simulink model "bh_3d_pend_sim_CONTROLLED"  (R2021b)
settings: Solver=ode45  StartTime=0.0  StopTime=25  FixedStep=0.001  RelTol=1e-6  AbsTol=1e-6  EnableMultiTasking=on
values from neighbouring files (symbols this model uses):
  K_LAW = [-78.361088012 1.69049101304e-13 6.50451101042e-15 -1.63175637691e-13 78.361088012 1.28612744558e-13 -17.2276366633 -1.91362461096e-14 -9.31673797735e-15 8.02726907722e-14 -17.2276366633 -2.57973956871e-14 ... (39 elements, 3x13)]    [OLD_bh_CONT_DES_RESULTS.mat]    (also in bh_CONT_DES_RESULTS.mat = [-78.361088012 -5.38759787414e-13 -4.00721571005e-14 3.64954)
undefined symbols (not defined in the file or in its folder): DOT_Phi_Theta_Psi, DOT_XYZ, g, Hx, Hy, Hz, Lx, Ly, Lz, M_cart, m_pend, Phi_Theta_Psi, q0_ang_deg, q0_dot_and_deg, sigbuilder_block, X, XYZ, Y, Z
libraries: nesl_utility x14, simulink_extras x11, sm_lib x9
(part 1 of 2)
settings Model: Creator=bhorton  LastModifiedBy=bhorton
settings SolverCC: ZeroCrossAlgorithm=Adaptive  AlgebraicLoopSolver=TrustRegion
settings DataIOCC: LimitDataPoints=on  ReturnWorkspaceOutputs=off
settings OptimizationCC: LifeSpan=inf
settings DebuggingCC: AllowSymbolicDim=off  PregeneratedLibrarySubsystemCodeDiagnostic=none  SFUnexpectedBacktrackingDiag=warning  SFNoUnconditionalDefaultTransitionDiag=warning  SFExecutionAtInitializationDiag=none  SFMachineParentedDataDiag=warning  ArithmeticOperatorsInVariantConditions=warning
settings SFSimCC: SimUseLocalCustomCode=off  CustomCodeUndefinedFunction=UseInterfaceOnly
settings RTWCC: RTWUseLocalCustomCode=off
settings CodeAppCC: StateflowObjectComments=on
settings GRTTargetCC: TargetLangStandard=C89/C90 (ANSI)
settings ConfigComp: CovMetricSettings=dw  CovSaveCumulativeToWorkspaceVar=on  CovSaveSingleToWorkspaceVar=on  CovExternalEMLEnable=off  CovSFcnEnable=off
settings SimscapeCC: SimscapeNormalizeSystem=off  SimscapeLogType=all  SimscapeLogDataHistory=10000
settings ConfigurationSet: Description=SimMechanics 2G
settings ExplorerConfigSet: InternalSimMechanicsExplorerSettings="<ExplorerConfiguration><canonicalview>default</canonicalview><AnimationSetting><BasePlaybackSpeed>1.0</BasePlaybackSpeed><PlaybackSpeedFactor>1.0</PlaybackSpeedFactor></AnimationSetting><TilePanel><TileInfo><Tiles Columns=\"2\" Count=\"4\" Rows=\"2\"><Column Left=\"2\" Weight=\"0.4993\"/><Column Left=\"299\" Weight=\"0.5007\"/><Column Left=\"596\"/><Row Top=\"2\" Weight=\"0.4991\"/><Row Top=\"230\" Weight=\"0.5009\"/><Row Top=\"459\"/><Tile Height=\"1\" Width=\"1\" X=\"0\" Y=\"0\"/><Tile Height=\"1\" Width=\"1\" X=\"0\" Y=\"1\"/><Tile Height=\"1\" Width=\"1\" X=\"1\" Y=\"0\"/><Tile Height=\"1\" Width=\"1\" X=\"1\" Y=\"1\"/></Tiles></TileInfo><SceneInfo><SceneViewer><BGColor><R>0.60000002384185791</R><G>0.60000002384185791</G><B>0.60000002384185791</B></BGColor><Camera><DoPerspective>off</DoPerspective><Position><X>0.0066101237906532632</X><Y>-1.0000000187716092</Y><Z>0.27830506136231026</Z></Position><Center><X>0.0066101237906532632</X><Y>-1.8771609211487572e-08</Y><Z>0.27830506136231026</Z></Center><Up><X>0</X><Y>-0</Y><Z>1</Z></Up><ViewLimDist>1</ViewLimDist><YLim>0.6337593571276271</YLim><XLim>0.8334369627979753</XLim></Camera></SceneViewer><SceneViewer><BGColor><R>0.60000002384185791</R><G>0.60000002384185791</G><B>0.60000002384185791</B></BGColor><Camera><DoPerspective>off</DoPerspective><Position><X>0.12097194898226168</X><Y>-0.1831262202380439</Y><Z>1.2750000010896152</Z></Position><Center><X>0.12097194898226168</X><Y>-0.1831262202380439</Y><Z>0.2750000010896152</Z></Center><Up><X>0</X><Y>1</Y><Z>-0</Z></Up><ViewLimDist>1</ViewLimDist><YLim>0.56280693766119472</YLim><XLim>0.73676544566556401</XLim></Camera></SceneViewer><SceneViewer><BGColor><R>0.60000002384185791</R><G>0.60000002384185791</G><B>0.60000002384185791</B></BGColor><Camera><DoPerspective>off</DoPerspective><Position><X>1.0477103451195624</X><Y>0.043433240975990085</Y><Z>0.24150487446228938</Z></Position><Center><X>3.245263613393945e-09</X><Y>0.043433240975990085</Y><Z>0.24150487446228938</Z></Center><Up><X>-0</X><Y>0</Y><Z>1</Z></Up><ViewLimDist>1</ViewLimDist><YLim>0.53585596018430881</YLim><XLim>0.70468729010539233</XLim></Camera></SceneViewer><SceneViewer><BGColor><R>0.60000002384185791</R><G>0.60000002384185791</G><B>0.60000002384185791</B></BGColor><Camera><DoPerspective>off</DoPerspective><Position><X>0.62223409931486595</X><Y>-0.53029272300920749</Y><Z>0.80202361126646926</Z></Position><Center><X>0.044883830125240165</X><Y>0.047057546180418207</Y><Z>0.2246733420768435</Z></Center><Up><X>-0.40824829046386307</X><Y>0.40824829046386307</Y><Z>0.81649658092772615</Z></Up><ViewLimDist>1</ViewLimDist><YLim>0.76349703631239541</YLim><XLim>0.99948702935440847</XLim></Camera></SceneViewer></SceneInfo></TilePanel><MechEditorPanel><Cameras/><GfxPanelCameraMap/><VideoCreator><PlaybackSpeedRatio>1.0</PlaybackSpeedRatio><FrameRate>30</FrameRate><VideoFormat>Motion JPEG AVI</VideoFormat><FrameSize>auto</FrameSize></VideoCreator></MechEditorPanel></ExplorerConfiguration>"

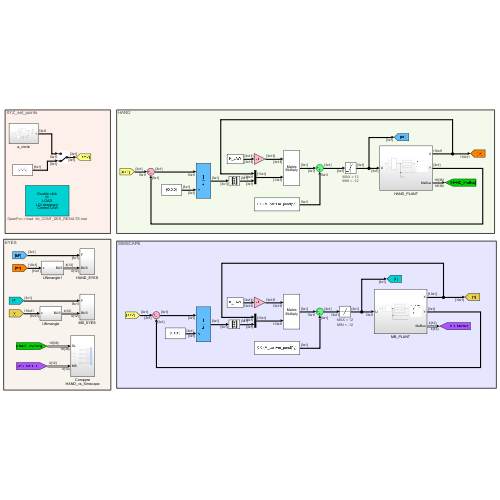
[thumbnail: Simulink's stored preview of the top-level diagram]
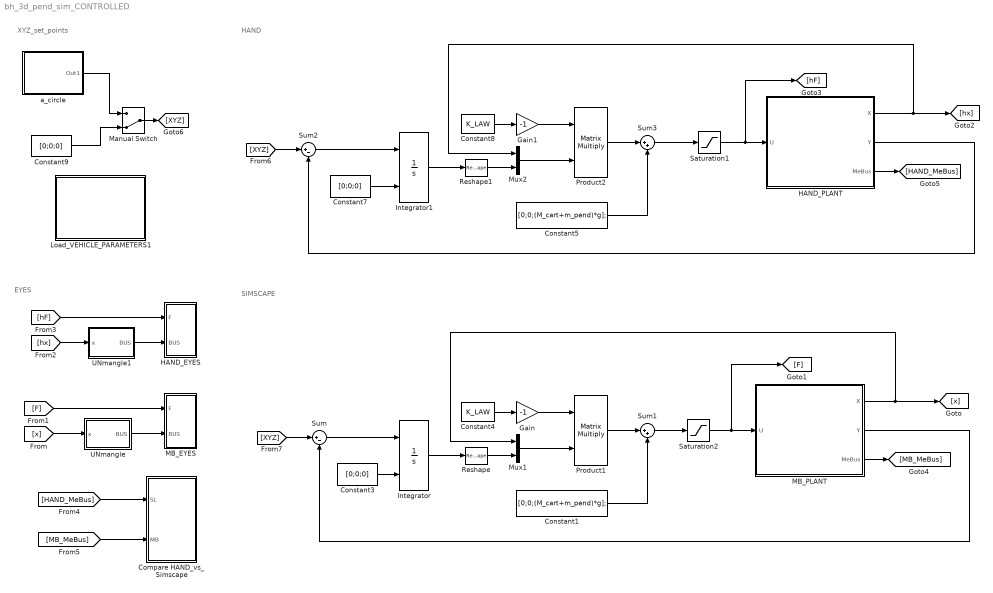
== system bh_3d_pend_sim_CONTROLLED ==
  note: XYZ_set_points
  note: EYES
  note: HAND
  note: SIMSCAPE
  Compare HAND_vs_Simscape : Subsystem
  Constant1 : Constant  Value=[0;0;(M_cart+m_pend)*g];  VectorParams1D=off
  Constant3 : Constant  Value=[0;0;0]  VectorParams1D=off
  Constant4 : Constant  Value=K_LAW  VectorParams1D=off
  Constant5 : Constant  Value=[0;0;(M_cart+m_pend)*g];  VectorParams1D=off
  Constant7 : Constant  Value=[0;0;0]  VectorParams1D=off
  Constant8 : Constant  Value=K_LAW  VectorParams1D=off
  Constant9 : Constant  Value=[0;0;0]  VectorParams1D=off
  Gain : Gain  Gain=-1
  Gain1 : Gain  Gain=-1
  HAND_EYES : Subsystem
  HAND_PLANT : Subsystem
  Integrator : Integrator  InitialConditionSource=external
  Integrator1 : Integrator  InitialConditionSource=external
  Load_VEHICLE_PARAMETERS1 : Subsystem
      settings: AttributesFormatString=OpenFcn = %<OpenFcn>  OpenFcn="load  bh_CONT_DES_RESULTS.mat"
      mask Display: disp('Double click\nto\nLOAD\nLQI designed \n Control LAW')
  MB_EYES : Subsystem
  MB_PLANT : Subsystem
  Manual Switch : ManualSwitch  CurrentSetting=0
  Mux1 : Mux  Inputs=2
  Mux2 : Mux  Inputs=2
  Product1 : Product  Multiplication=Matrix(*)
  Product2 : Product  Multiplication=Matrix(*)
  Reshape : Reshape  OutputDimensionality=Column vector (2-D)
  Reshape1 : Reshape  OutputDimensionality=Column vector (2-D)
  Saturation1 : Saturate  UpperLimit=12  LowerLimit=-12
      settings: AttributesFormatString=|
      | MAX = %<UpperLimit>
      | MIN = %<LowerLimit>
  Saturation2 : Saturate  UpperLimit=12  LowerLimit=-12
      settings: AttributesFormatString=|
      | MAX = %<UpperLimit>
      | MIN = %<LowerLimit>
  Sum : Sum  Inputs=|+-
  Sum1 : Sum  Inputs=|++
  Sum2 : Sum  Inputs=|+-
  Sum3 : Sum  Inputs=|++
  UNmangle : Subsystem
  UNmangle1 : Subsystem
  a_circle : Subsystem
  wires:
  Mux1/1 -> Product1/2
  Integrator/1 -> Reshape/1
  MB_PLANT/2(Y) -> Sum/2
  Constant3/1 -> Integrator/2
  Product1/1 -> Sum1/1
  Gain/1 -> Product1/1
  Sum/1 -> Integrator/1
  MB_PLANT/1(X) -> [x], Mux1/1
  [XYZ] -> Sum/1
  Constant4/1 -> Gain/1
  Reshape/1 -> Mux1/2
  [F] -> MB_EYES/1(F)
  UNmangle/1(BUS) -> MB_EYES/2(BUS)
  [x] -> UNmangle/1(x)
  Saturation2/1 -> [F], MB_PLANT/1(U)
  Sum1/1 -> Saturation2/1
  Constant1/1 -> Sum1/2
  Saturation1/1 -> [hF], HAND_PLANT/1(U)
  Gain1/1 -> Product2/1
  Constant7/1 -> Integrator1/2
  Sum3/1 -> Saturation1/1
  Sum2/1 -> Integrator1/1
  [XYZ] -> Sum2/1
  HAND_PLANT/2(Y) -> Sum2/2
  Mux2/1 -> Product2/2
  Integrator1/1 -> Reshape1/1
  Product2/1 -> Sum3/1
  Reshape1/1 -> Mux2/2
  Constant5/1 -> Sum3/2
  Constant8/1 -> Gain1/1
  HAND_PLANT/1(X) -> [hx], Mux2/1
  UNmangle1/1(BUS) -> HAND_EYES/2(BUS)
  [hx] -> UNmangle1/1(x)
  [hF] -> HAND_EYES/1(F)
  [HAND_MeBus] -> Compare HAND_vs_Simscape/1(SL)
  [MB_MeBus] -> Compare HAND_vs_Simscape/2(MB)
  HAND_PLANT/3(MeBus) -> [HAND_MeBus]
  MB_PLANT/3(MeBus) -> [MB_MeBus]
  a_circle/1(Out1) -> Manual Switch/1
  Constant9/1 -> Manual Switch/2
  Manual Switch/1 -> [XYZ]

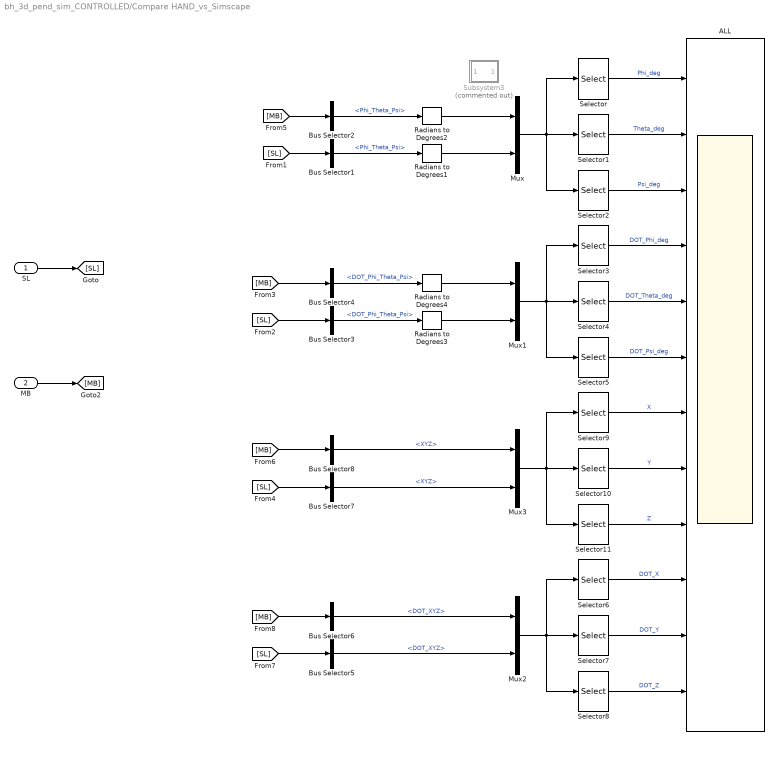
== system bh_3d_pend_sim_CONTROLLED/Compare HAND_vs_Simscape ==
  SL : Inport
  MB : Inport  Port=2
  ALL : Scope  NumInputPorts=12
  Bus Selector1 : BusSelector  OutputSignals=Phi_Theta_Psi
  Bus Selector2 : BusSelector  OutputSignals=Phi_Theta_Psi
  Bus Selector3 : BusSelector  OutputSignals=DOT_Phi_Theta_Psi
  Bus Selector4 : BusSelector  OutputSignals=DOT_Phi_Theta_Psi
  Bus Selector5 : BusSelector  OutputSignals=DOT_XYZ
  Bus Selector6 : BusSelector  OutputSignals=DOT_XYZ
  Bus Selector7 : BusSelector  OutputSignals=XYZ
  Bus Selector8 : BusSelector  OutputSignals=XYZ
  Mux{,1..3} (4 alike) : Mux  Inputs=2
  Radians to Degrees{1..4} (4 alike) : simulink_extras/Transformations/Radians to Degrees
  Selector{,3,6,9} (4 alike) : Selector  InputPortWidth=6  IndexOptions=Index vector (dialog)  Indices=[1 4]  OutputSizes=1
  Selector{1,4,7,10} (4 alike) : Selector  InputPortWidth=6  IndexOptions=Index vector (dialog)  Indices=[2 5]  OutputSizes=1
  Selector{2,5,8,11} (4 alike) : Selector  InputPortWidth=6  IndexOptions=Index vector (dialog)  Indices=[3 6]  OutputSizes=1
  Subsystem3 : Subsystem  Commented=on
      mask Display: disp(sprintf('Mod\n360'))
  wires:
  SL/1 -> [SL]
  MB/1 -> [MB]
  Bus Selector1/1 -> Radians to Degrees1/1  "<Phi_Theta_Psi>"
  Bus Selector2/1 -> Radians to Degrees2/1  "<Phi_Theta_Psi>"
  Radians to Degrees1/1 -> Mux/2
  Radians to Degrees2/1 -> Mux/1
  Selector/1 -> ALL/1  "Phi_deg"
  Selector2/1 -> ALL/3  "Psi_deg"
  Selector1/1 -> ALL/2  "Theta_deg"
  Mux/1 -> Selector2/1, Selector/1, Selector1/1
  Bus Selector3/1 -> Radians to Degrees3/1  "<DOT_Phi_Theta_Psi>"
  Radians to Degrees3/1 -> Mux1/2
  Bus Selector4/1 -> Radians to Degrees4/1  "<DOT_Phi_Theta_Psi>"
  Radians to Degrees4/1 -> Mux1/1
  Mux1/1 -> Selector5/1, Selector3/1, Selector4/1
  Selector4/1 -> ALL/5  "DOT_Theta_deg"
  Selector3/1 -> ALL/4  "DOT_Phi_deg"
  Selector5/1 -> ALL/6  "DOT_Psi_deg"
  Mux2/1 -> Selector8/1, Selector6/1, Selector7/1
  Bus Selector6/1 -> Mux2/1  "<DOT_XYZ>"
  Bus Selector5/1 -> Mux2/2  "<DOT_XYZ>"
  Selector7/1 -> ALL/11  "DOT_Y"
  Selector8/1 -> ALL/12  "DOT_Z"
  Selector6/1 -> ALL/10  "DOT_X"
  Bus Selector7/1 -> Mux3/2  "<XYZ>"
  Bus Selector8/1 -> Mux3/1  "<XYZ>"
  Mux3/1 -> Selector11/1, Selector9/1, Selector10/1
  Selector9/1 -> ALL/7  "X"
  Selector10/1 -> ALL/8  "Y"
  Selector11/1 -> ALL/9  "Z"
  [MB] -> Bus Selector2/1
  [SL] -> Bus Selector1/1
  [MB] -> Bus Selector6/1
  [SL] -> Bus Selector5/1
  [SL] -> Bus Selector7/1
  [MB] -> Bus Selector8/1
  [SL] -> Bus Selector3/1
  [MB] -> Bus Selector4/1

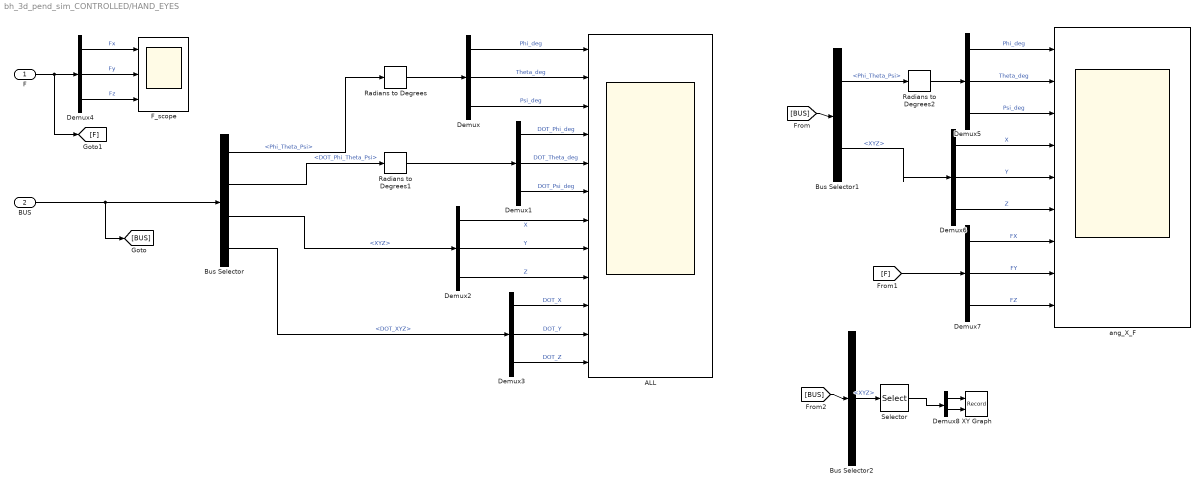
== system bh_3d_pend_sim_CONTROLLED/HAND_EYES ==
  F : Inport
  BUS : Inport  Port=2
  ALL : Scope  NumInputPorts=12
  Bus Selector : BusSelector  OutputSignals=Phi_Theta_Psi,DOT_Phi_Theta_Psi,XYZ,DOT_XYZ
  Bus Selector1 : BusSelector  OutputSignals=Phi_Theta_Psi,XYZ
  Bus Selector2 : BusSelector  OutputSignals=XYZ
  Demux{,1..7} (8 alike) : Demux  Outputs=3
  Demux8 : Demux  Outputs=2
  F_scope : Scope  NumInputPorts=3
  Radians to Degrees : simulink_extras/Transformations/Radians to Degrees
  Radians to Degrees1 : simulink_extras/Transformations/Radians to Degrees
  Radians to Degrees2 : simulink_extras/Transformations/Radians to Degrees
  Selector : Selector  InputPortWidth=3  IndexOptions=Index vector (dialog)  Indices=[1 2]  OutputSizes=1
  XY Graph : Record  FileSettingsInternal="{\"entries\":[{\"content\":{\"excelSettings\":{\"content\":{},\"type\":\"Streamout.ExcelSettings\"}},\"type\":\"Streamout.FileSettingStorage\",\"uuid\":\"99c117ed-58ae-4b65-b485-cface1eea5be\"}],\"packageUris\":[\"http://schema.mathworks.com/mf0/streamout_blocks/R2020a\"],\"version\":\"1.0\"}"  Layout=[1 1]  SignalsInternal="{\"entries\":[{\"content\":{\"signals\":[{\"content\":{\"blockPath\":[\"bh_3d_pend_sim_CONTROLLED/HAND_EYES/XY Graph\"],\"channel\":[],\"dimensions\":[1,1],\"domain\":\"bh_3d_pend_sim_CONTROLLED/HAND_EYES/XY Graph\",\"lineColor\":\"#a2142f\",\"plots\":[1],\"port\":1,\"sid\":[\"\"],\"signalID\":34,\"signalName\":\"Demux8:1\"},\"type\":\"RecordBlkView.Signal\",\"uuid\":\"b9760cf6-ac66-4326-8e3b-6ee9031ad026\"},{\"content\":{\"blockPath\":[\"bh_3d_pend_sim_CONTROLLED/HAND_EYES/XY Graph\"],\"channel\":[],\"dimensions\":[1,1],\"domain\":\"bh_3d_pend_sim_CONTROLLED/HAND_EYES/XY Graph\",\"lineColor\":\"#139fff\",\"plots\":[1],\"port\":2,\"sid\":[\"\"],\"signalID\":38,\"signalName\":\"Demux8:2\"},\"type\":\"RecordBlkView.Signal\",\"uuid\":\"94cb77a1-340e-480f-8b2e-a2f08ce9c347\"}]},\"type\":\"RecordBlkView.InputSignals\",\"uuid\":\"3dd7e1b0-0053-45f3-aee9-dc3925895e13\"}],\"packageUris\":[\"http://schema.mathworks.com/mf0/streamout_blocks/R2020a\"],\"version\":\"1.0\"}"  VisualizationBindings="{\"xyplotplugin\":{\"info\":[{\"series\":[{\"bindingParametersList\":[{\"parameter\":\"X-Axis\",\"signalID\":34,\"signalName\":\"Demux8:1\"},{\"parameter\":\"Y-Axis\",\"signalID\":38,\"signalName\":\"Demux8:2\"}],\"seriesID\":54278}],\"subplotID\":1}]}}"  CompatibilityTag=XY  st=-1
  ang_X_F : Scope  NumInputPorts=9
  wires:
  Bus Selector/2 -> Radians to Degrees1/1  "<DOT_Phi_Theta_Psi>"
  Bus Selector/1 -> Radians to Degrees/1  "<Phi_Theta_Psi>"
  Demux4/3 -> F_scope/3  "Fz"
  Demux4/1 -> F_scope/1  "Fx"
  Demux/1 -> ALL/1  "Phi_deg"
  Radians to Degrees1/1 -> Demux1/1
  Demux3/3 -> ALL/12  "DOT_Z"
  Demux1/3 -> ALL/6  "DOT_Psi_deg"
  Bus Selector/3 -> Demux2/1  "<XYZ>"
  Demux3/1 -> ALL/10  "DOT_X"
  Demux2/3 -> ALL/9  "Z"
  Demux3/2 -> ALL/11  "DOT_Y"
  Demux2/2 -> ALL/8  "Y"
  Demux2/1 -> ALL/7  "X"
  Demux1/1 -> ALL/4  "DOT_Phi_deg"
  Demux1/2 -> ALL/5  "DOT_Theta_deg"
  Demux/2 -> ALL/2  "Theta_deg"
  BUS/1 -> [BUS], Bus Selector/1
  Demux/3 -> ALL/3  "Psi_deg"
  Bus Selector/4 -> Demux3/1  "<DOT_XYZ>"
  Radians to Degrees/1 -> Demux/1
  Demux4/2 -> F_scope/2  "Fy"
  F/1 -> [F], Demux4/1
  [BUS] -> Bus Selector1/1
  Bus Selector1/1 -> Radians to Degrees2/1  "<Phi_Theta_Psi>"
  Demux5/3 -> ang_X_F/3  "Psi_deg"
  Demux5/2 -> ang_X_F/2  "Theta_deg"
  Demux5/1 -> ang_X_F/1  "Phi_deg"
  Radians to Degrees2/1 -> Demux5/1
  Demux6/1 -> ang_X_F/4  "X"
  Demux6/2 -> ang_X_F/5  "Y"
  Demux6/3 -> ang_X_F/6  "Z"
  Bus Selector1/2 -> Demux6/1  "<XYZ>"
  Demux7/1 -> ang_X_F/7  "FX"
  Demux7/2 -> ang_X_F/8  "FY"
  [F] -> Demux7/1
  Demux7/3 -> ang_X_F/9  "FZ"
  [BUS] -> Bus Selector2/1
  Demux8/1 -> XY Graph/1
  Demux8/2 -> XY Graph/2
  Bus Selector2/1 -> Selector/1  "<XYZ>"
  Selector/1 -> Demux8/1

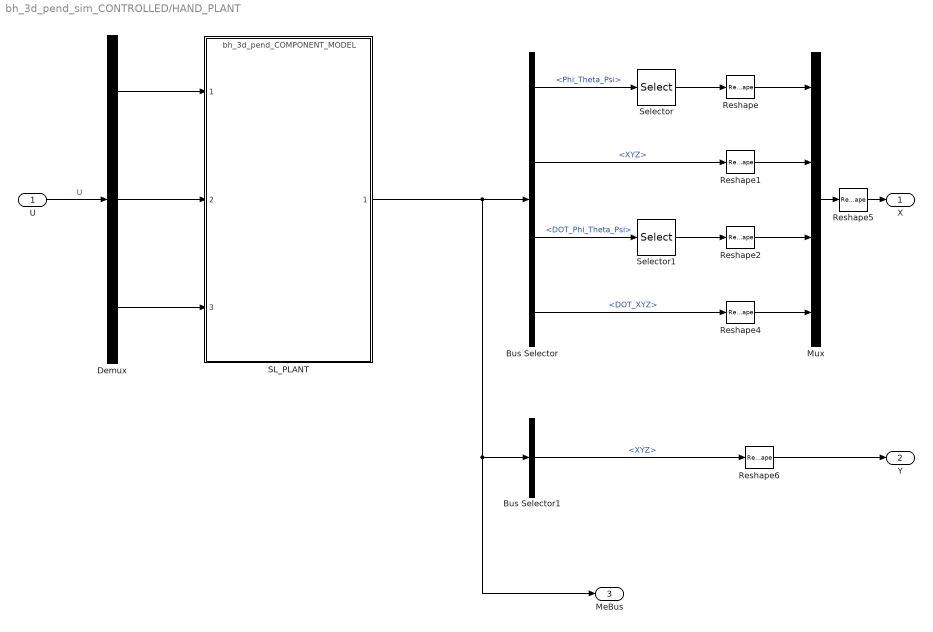
== system bh_3d_pend_sim_CONTROLLED/HAND_PLANT ==
  U : Inport
  Bus Selector : BusSelector  OutputSignals=Phi_Theta_Psi,XYZ,DOT_Phi_Theta_Psi,DOT_XYZ
  Bus Selector1 : BusSelector  OutputSignals=XYZ
  Demux : Demux  Outputs=3
  Mux : Mux
  Reshape{,1..2,4..6} (6 alike) : Reshape  OutputDimensionality=Column vector (2-D)
  SL_PLANT : ModelReference  ModelNameDialog=bh_3d_pend_COMPONENT_MODEL.slx  SimulationMode=Normal  ModelReferenceVersion=5.0
  Selector : Selector  InputPortWidth=3  IndexOptions=Index vector (dialog)  Indices=2:3  OutputSizes=1
  Selector1 : Selector  InputPortWidth=3  IndexOptions=Index vector (dialog)  Indices=2:3  OutputSizes=1
  X : Outport  VectorParamsAs1DForOutWhenUnconnected=off
  Y : Outport  Port=2  VectorParamsAs1DForOutWhenUnconnected=off
  MeBus : Outport  Port=3  VectorParamsAs1DForOutWhenUnconnected=off
  wires:
  Demux/1 -> SL_PLANT/1
  Demux/2 -> SL_PLANT/2
  Demux/3 -> SL_PLANT/3
  U/1 -> Demux/1  "U"
  SL_PLANT/1 -> MeBus/1, Bus Selector1/1, Bus Selector/1
  Bus Selector/1 -> Selector/1  "<Phi_Theta_Psi>"
  Bus Selector/2 -> Reshape1/1  "<XYZ>"
  Bus Selector/3 -> Selector1/1  "<DOT_Phi_Theta_Psi>"
  Selector1/1 -> Reshape2/1
  Selector/1 -> Reshape/1
  Bus Selector/4 -> Reshape4/1  "<DOT_XYZ>"
  Reshape2/1 -> Mux/3
  Reshape1/1 -> Mux/2
  Reshape/1 -> Mux/1
  Reshape4/1 -> Mux/4
  Mux/1 -> Reshape5/1
  Reshape5/1 -> X/1
  Reshape6/1 -> Y/1
  Bus Selector1/1 -> Reshape6/1  "<XYZ>"

== system bh_3d_pend_sim_CONTROLLED/Load_VEHICLE_PARAMETERS1 ==

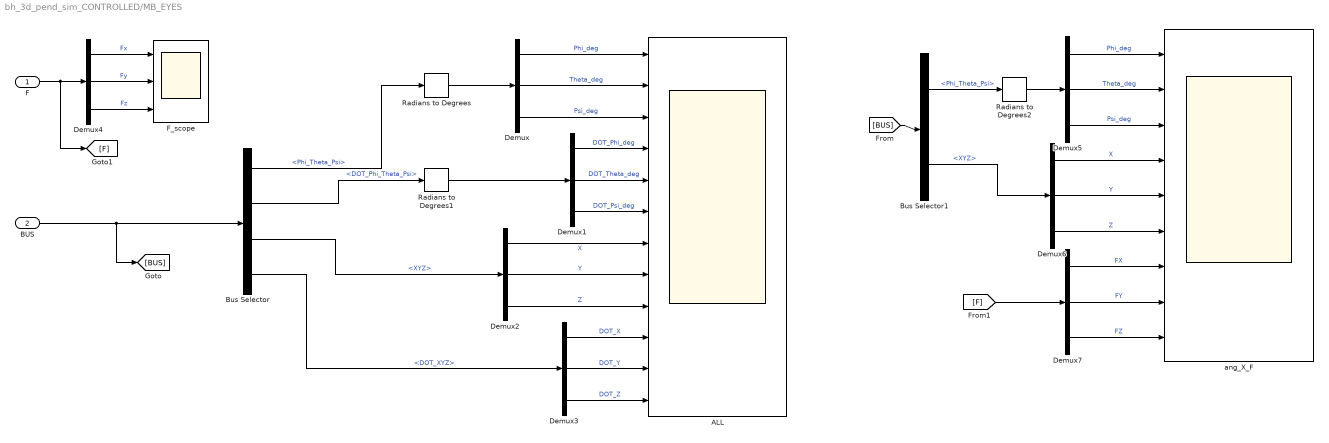
== system bh_3d_pend_sim_CONTROLLED/MB_EYES ==
  F : Inport
  BUS : Inport  Port=2
  ALL : Scope  NumInputPorts=12
  Bus Selector : BusSelector  OutputSignals=Phi_Theta_Psi,DOT_Phi_Theta_Psi,XYZ,DOT_XYZ
  Bus Selector1 : BusSelector  OutputSignals=Phi_Theta_Psi,XYZ
  Demux{,1..7} (8 alike) : Demux  Outputs=3
  F_scope : Scope  NumInputPorts=3
  Radians to Degrees : simulink_extras/Transformations/Radians to Degrees
  Radians to Degrees1 : simulink_extras/Transformations/Radians to Degrees
  Radians to Degrees2 : simulink_extras/Transformations/Radians to Degrees
  ang_X_F : Scope  NumInputPorts=9
  wires:
  Bus Selector/2 -> Radians to Degrees1/1  "<DOT_Phi_Theta_Psi>"
  Bus Selector/1 -> Radians to Degrees/1  "<Phi_Theta_Psi>"
  Demux4/3 -> F_scope/3  "Fz"
  Demux4/1 -> F_scope/1  "Fx"
  Demux/1 -> ALL/1  "Phi_deg"
  Radians to Degrees1/1 -> Demux1/1
  Demux3/3 -> ALL/12  "DOT_Z"
  Demux1/3 -> ALL/6  "DOT_Psi_deg"
  Bus Selector/3 -> Demux2/1  "<XYZ>"
  Demux3/1 -> ALL/10  "DOT_X"
  Demux2/3 -> ALL/9  "Z"
  Demux3/2 -> ALL/11  "DOT_Y"
  Demux2/2 -> ALL/8  "Y"
  Demux2/1 -> ALL/7  "X"
  Demux1/1 -> ALL/4  "DOT_Phi_deg"
  Demux1/2 -> ALL/5  "DOT_Theta_deg"
  Demux/2 -> ALL/2  "Theta_deg"
  BUS/1 -> [BUS], Bus Selector/1
  Demux/3 -> ALL/3  "Psi_deg"
  Bus Selector/4 -> Demux3/1  "<DOT_XYZ>"
  Radians to Degrees/1 -> Demux/1
  Demux4/2 -> F_scope/2  "Fy"
  F/1 -> [F], Demux4/1
  [BUS] -> Bus Selector1/1
  Bus Selector1/1 -> Radians to Degrees2/1  "<Phi_Theta_Psi>"
  Demux5/3 -> ang_X_F/3  "Psi_deg"
  Demux5/2 -> ang_X_F/2  "Theta_deg"
  Demux5/1 -> ang_X_F/1  "Phi_deg"
  Radians to Degrees2/1 -> Demux5/1
  Demux6/1 -> ang_X_F/4  "X"
  Demux6/2 -> ang_X_F/5  "Y"
  Demux6/3 -> ang_X_F/6  "Z"
  Bus Selector1/2 -> Demux6/1  "<XYZ>"
  Demux7/1 -> ang_X_F/7  "FX"
  Demux7/2 -> ang_X_F/8  "FY"
  [F] -> Demux7/1
  Demux7/3 -> ang_X_F/9  "FZ"

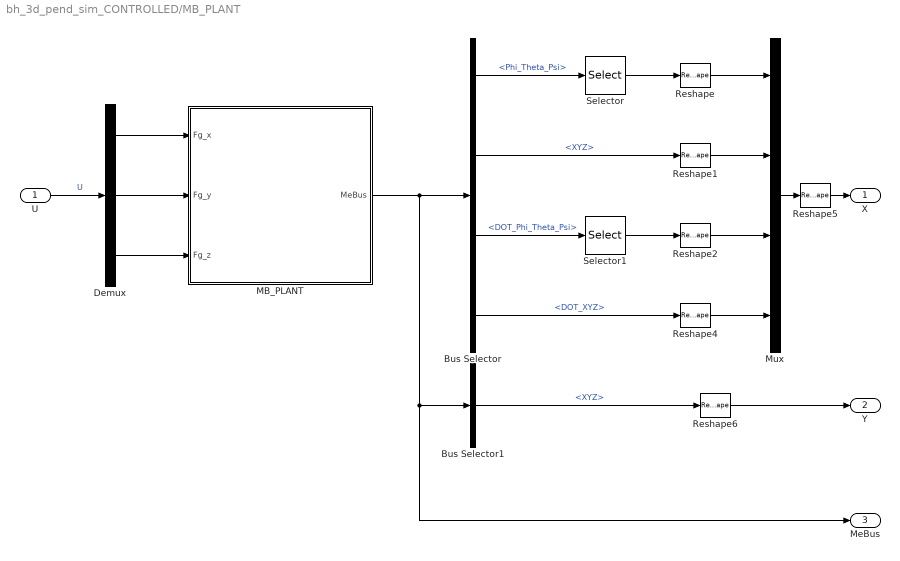
== system bh_3d_pend_sim_CONTROLLED/MB_PLANT ==
  U : Inport
  Bus Selector : BusSelector  OutputSignals=Phi_Theta_Psi,XYZ,DOT_Phi_Theta_Psi,DOT_XYZ
  Bus Selector1 : BusSelector  OutputSignals=XYZ
  Demux : Demux  Outputs=3
  MB_PLANT : Subsystem
  Mux : Mux
  Reshape{,1..2,4..6} (6 alike) : Reshape  OutputDimensionality=Column vector (2-D)
  Selector : Selector  InputPortWidth=3  IndexOptions=Index vector (dialog)  Indices=2:3  OutputSizes=1
  Selector1 : Selector  InputPortWidth=3  IndexOptions=Index vector (dialog)  Indices=2:3  OutputSizes=1
  X : Outport  VectorParamsAs1DForOutWhenUnconnected=off
  Y : Outport  Port=2  VectorParamsAs1DForOutWhenUnconnected=off
  MeBus : Outport  Port=3  VectorParamsAs1DForOutWhenUnconnected=off
  wires:
  Demux/1 -> MB_PLANT/1(Fg_x)
  Demux/2 -> MB_PLANT/2(Fg_y)
  Demux/3 -> MB_PLANT/3(Fg_z)
  U/1 -> Demux/1  "U"
  MB_PLANT/1(MeBus) -> MeBus/1, Bus Selector1/1, Bus Selector/1
  Bus Selector/1 -> Selector/1  "<Phi_Theta_Psi>"
  Bus Selector/2 -> Reshape1/1  "<XYZ>"
  Bus Selector/3 -> Selector1/1  "<DOT_Phi_Theta_Psi>"
  Selector1/1 -> Reshape2/1
  Selector/1 -> Reshape/1
  Bus Selector/4 -> Reshape4/1  "<DOT_XYZ>"
  Reshape2/1 -> Mux/3
  Reshape1/1 -> Mux/2
  Reshape/1 -> Mux/1
  Reshape4/1 -> Mux/4
  Mux/1 -> Reshape5/1
  Reshape5/1 -> X/1
  Reshape6/1 -> Y/1
  Bus Selector1/1 -> Reshape6/1  "<XYZ>"

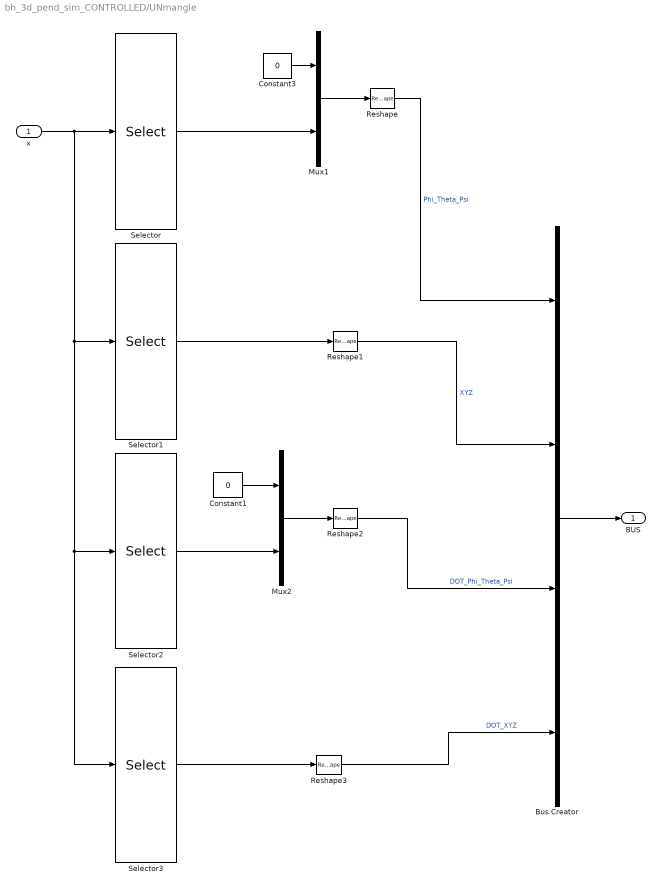
== system bh_3d_pend_sim_CONTROLLED/UNmangle ==
  x : Inport
  Bus Creator : BusCreator  Inputs=4
  Constant1 : Constant  Value=0  VectorParams1D=off
  Constant3 : Constant  Value=0  VectorParams1D=off
  Mux1 : Mux  Inputs=2
  Mux2 : Mux  Inputs=2
  Reshape{,1..3} (4 alike) : Reshape  OutputDimensionality=Column vector (2-D)
  Selector : Selector  InputPortWidth=10  IndexOptions=Index vector (dialog)  Indices=[1,2]  OutputSizes=1
  Selector1 : Selector  InputPortWidth=10  IndexOptions=Index vector (dialog)  Indices=3:5  OutputSizes=1
  Selector2 : Selector  InputPortWidth=10  IndexOptions=Index vector (dialog)  Indices=6:7  OutputSizes=1
  Selector3 : Selector  InputPortWidth=10  IndexOptions=Index vector (dialog)  Indices=8:10  OutputSizes=1
  BUS : Outport  VectorParamsAs1DForOutWhenUnconnected=off
  wires:
  x/1 -> Selector3/1, Selector2/1, Selector1/1, Selector/1
  Constant3/1 -> Mux1/1
  Selector/1 -> Mux1/2
  Mux1/1 -> Reshape/1
  Selector1/1 -> Reshape1/1
  Selector2/1 -> Mux2/2
  Constant1/1 -> Mux2/1
  Mux2/1 -> Reshape2/1
  Selector3/1 -> Reshape3/1
  Bus Creator/1 -> BUS/1
  Reshape/1 -> Bus Creator/1  "Phi_Theta_Psi"
  Reshape1/1 -> Bus Creator/2  "XYZ"
  Reshape2/1 -> Bus Creator/3  "DOT_Phi_Theta_Psi"
  Reshape3/1 -> Bus Creator/4  "DOT_XYZ"

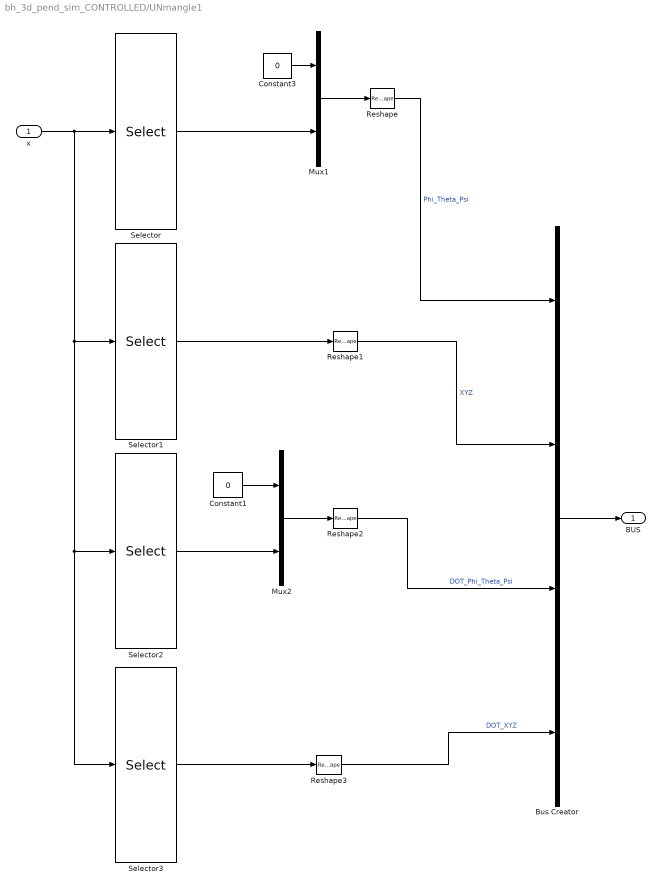
== system bh_3d_pend_sim_CONTROLLED/UNmangle1 ==
  x : Inport
  Bus Creator : BusCreator  Inputs=4
  Constant1 : Constant  Value=0  VectorParams1D=off
  Constant3 : Constant  Value=0  VectorParams1D=off
  Mux1 : Mux  Inputs=2
  Mux2 : Mux  Inputs=2
  Reshape{,1..3} (4 alike) : Reshape  OutputDimensionality=Column vector (2-D)
  Selector : Selector  InputPortWidth=10  IndexOptions=Index vector (dialog)  Indices=[1,2]  OutputSizes=1
  Selector1 : Selector  InputPortWidth=10  IndexOptions=Index vector (dialog)  Indices=3:5  OutputSizes=1
  Selector2 : Selector  InputPortWidth=10  IndexOptions=Index vector (dialog)  Indices=6:7  OutputSizes=1
  Selector3 : Selector  InputPortWidth=10  IndexOptions=Index vector (dialog)  Indices=8:10  OutputSizes=1
  BUS : Outport  VectorParamsAs1DForOutWhenUnconnected=off
  wires:
  x/1 -> Selector3/1, Selector2/1, Selector1/1, Selector/1
  Constant3/1 -> Mux1/1
  Selector/1 -> Mux1/2
  Mux1/1 -> Reshape/1
  Selector1/1 -> Reshape1/1
  Selector2/1 -> Mux2/2
  Constant1/1 -> Mux2/1
  Mux2/1 -> Reshape2/1
  Selector3/1 -> Reshape3/1
  Bus Creator/1 -> BUS/1
  Reshape/1 -> Bus Creator/1  "Phi_Theta_Psi"
  Reshape1/1 -> Bus Creator/2  "XYZ"
  Reshape2/1 -> Bus Creator/3  "DOT_Phi_Theta_Psi"
  Reshape3/1 -> Bus Creator/4  "DOT_XYZ"

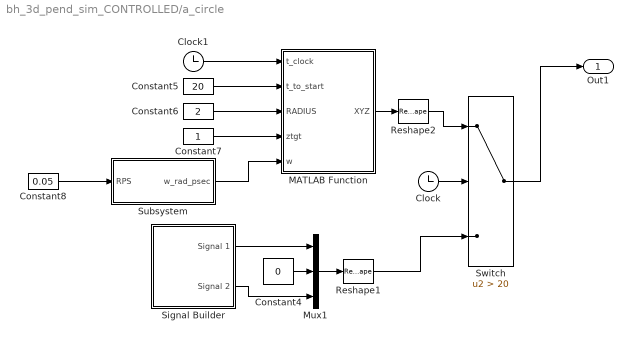
== system bh_3d_pend_sim_CONTROLLED/a_circle ==
  Clock : Clock
  Clock1 : Clock
  Constant4 : Constant  Value=0  VectorParams1D=off
  Constant5 : Constant  Value=20  VectorParams1D=off
  Constant6 : Constant  Value=2  VectorParams1D=off
  Constant7 : Constant  VectorParams1D=off
  Constant8 : Constant  Value=0.05  VectorParams1D=off
  MATLAB Function : MATLAB Function  TreatAsAtomicUnit=on
  Mux1 : Mux  Inputs=3
  Reshape1 : Reshape  OutputDimensionality=Column vector (2-D)
  Reshape2 : Reshape  OutputDimensionality=Column vector (2-D)
  Signal Builder : Subsystem  Tag=STV Subsys  LoadFcn=sigbuilder_block('load');  StartFcn=sigbuilder_block('start');  StopFcn=sigbuilder_block('stop');  ClipboardFcn=sigbuilder_block('clipboard');  mask(Sigbuilder block){tuvar=[0:10]}
      mask help: Simulink:masks:SigbuilderBlock_MD
      mask init:
      | if ~strcmp(get_param(bdroot(gcbh),'SimulationStatus'),'stopped') tuvar = sigbuilder_block('maskInit'); end
      settings: CopyFcn=sigbuilder_block('copy');  DeleteFcn=sigbuilder_block('delete');  ModelCloseFcn=sigbuilder_block('modelClose');  PreSaveFcn=sigbuilder_block('preSave');  PauseFcn=sigbuilder_block('pause');  ContinueFcn=sigbuilder_block('continue');  NameChangeFcn=sigbuilder_block('namechange');  OpenFcn=sigbuilder_block('open',[437.6 199.2 550.4 400 ]);  CloseFcn=sigbuilder_block('close');
      mask Display: plot(0, 0, 100, 100,[2, 2, 32, 32, 2], [68, 8, 8, 68, 68],[32, 2], [38, 38], [32, 19, 2],[53, 60, 44], [32, 17, 17, 2],[16, 16, 31, 31]);txt = getActiveGroup(gcbh);text(2, 100, txt,'verticalAlignment', 'top');
  Subsystem : Subsystem
  Switch : Switch  Criteria=u2 > Threshold  Threshold=20
  Out1 : Outport  VectorParamsAs1DForOutWhenUnconnected=off
  wires:
  Switch/1 -> Out1/1
  MATLAB Function/1(XYZ) -> Reshape2/1
  Constant6/1 -> MATLAB Function/3(RADIUS)
  Constant7/1 -> MATLAB Function/4(ztgt)
  Subsystem/1(w_rad_psec) -> MATLAB Function/5(w)
  Constant5/1 -> MATLAB Function/2(t_to_start)
  Reshape1/1 -> Switch/3
  Constant4/1 -> Mux1/2
  Signal Builder/1(Signal 1) -> Mux1/1
  Signal Builder/2(Signal 2) -> Mux1/3
  Mux1/1 -> Reshape1/1
  Clock/1 -> Switch/2
  Clock1/1 -> MATLAB Function/1(t_clock)
  Constant8/1 -> Subsystem/1(RPS)
  Reshape2/1 -> Switch/1

== system bh_3d_pend_sim_CONTROLLED/Compare HAND_vs_Simscape/Subsystem3 ==
  In1 : Inport
  Constant2 : Constant  Value=360
  Math Function : Math  Operator=mod  SignedPower=on  SaturateOnIntegerOverflow=on
  Out1 : Outport  VectorParamsAs1DForOutWhenUnconnected=off
  wires:
  Math Function/1 -> Out1/1
  In1/1 -> Math Function/1
  Constant2/1 -> Math Function/2

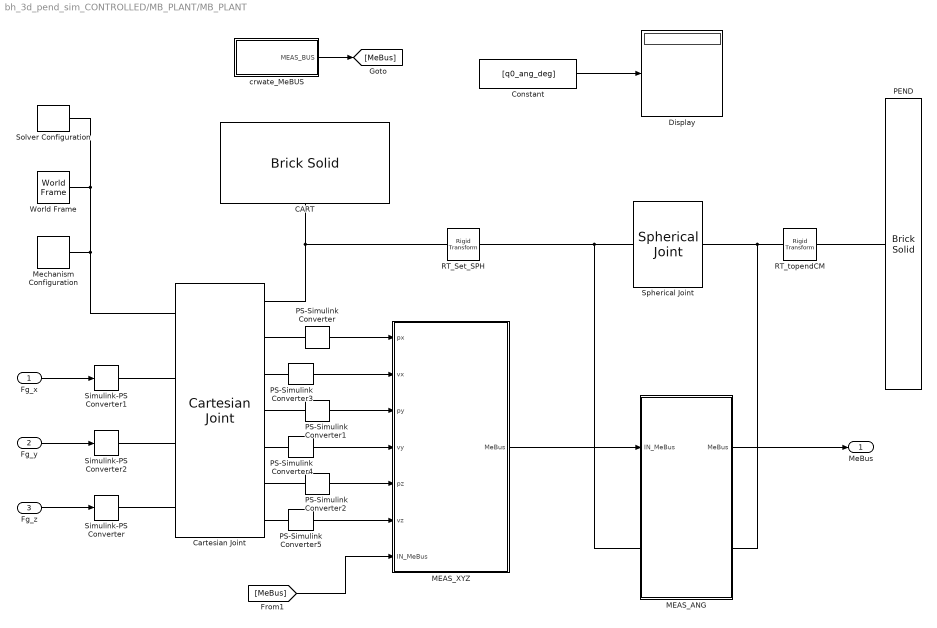
== system bh_3d_pend_sim_CONTROLLED/MB_PLANT/MB_PLANT ==
  Fg_x : Inport
  Fg_y : Inport  Port=2
  Fg_z : Inport  Port=3
  CART : sm_lib/Body Elements/Brick Solid  GraphicAmbientColor=[0.15 0.15 0.15 1.0]  BasedOnType=Mass  BrickDimensions=[Hx, Hy, Hz]  BrickDimensionUnits=m  CenterOfMass=[0 0 0]  CenterOfMassUnits=m  GraphicDiffuseColor=[0.2 0.2 1.0]  Density=1000  DensityUnits=kg/(m^3)  DoExposeReferenceFrame=on  GraphicEmissiveColor=[0.0 0.0 0.0 1.0]  ExportEntireGeometry=off  SerializedFrames=<Frames/>  MarkerShape=Sphere  MarkerSize=10  GraphicType=FromGeometry  InertiaType=PointMass  Mass=M_cart  MassUnits=kg  MomentsOfInertia=[1 1 1]  MomentsOfInertiaUnits=kg*m^2  GraphicOpacity=1.0  ProductsOfInertia=[0 0 0]  ProductsOfInertiaUnits=kg*m^2  GraphicShininess=75  GraphicSpecularColor=[0.5 0.5 0.5 1.0]  GraphicVisPropType=SimpleVisualProperties
  Cartesian Joint : sm_lib/Joints/Cartesian Joint  JointMode=Normal  SenseConstraintForce=off  SenseConstraintForceX=off  SenseConstraintForceY=off  SenseConstraintForceZ=off  SenseConstraintTorque=off  SenseConstraintTorqueX=off  SenseConstraintTorqueY=off  SenseConstraintTorqueZ=off  SenseTotalForce=off  SenseTotalForceX=off  SenseTotalForceY=off  SenseTotalForceZ=off  SenseTotalTorque=off  SenseTotalTorqueX=off  SenseTotalTorqueY=off  SenseTotalTorqueZ=off  CompositeWrenchDir=FollowerOnBase  CompositeWrenchFrame=BaseFrame  PxEquilibriumPosition=0  PxEquilibriumPositionUnits=m  PxSpringStiffness=0  PxSpringStiffnessUnits=N/m  PxDampingCoefficient=0  PxDampingCoefficientUnits=N/(m/s)  PxTorqueActuationMode=InputTorque  PxMotionActuationMode=ComputedMotion  PxSensePosition=on  PxSenseVelocity=on  PxSenseAcceleration=off  PxSenseTorqueForce=off  PxSenseLowerLimitTorqueForce=off  PxSenseUpperLimitTorqueForce=off  PxLowerLimitSpecify=off  PxLowerLimitBound=-1  PxLowerLimitBoundUnits=m  PxLowerLimitStiffness=1e6  PxLowerLimitStiffnessUnits=N/m  PxLowerLimitDamping=1e3  PxLowerLimitDampingUnits=N/(m/s)  PxLowerLimitTransitionRegionWidth=1e-4  PxLowerLimitTransitionRegionWidthUnits=m  PxUpperLimitSpecify=off  PxUpperLimitBound=1  PxUpperLimitBoundUnits=m  PxUpperLimitStiffness=1e6  PxUpperLimitStiffnessUnits=N/m  PxUpperLimitDamping=1e3  PxUpperLimitDampingUnits=N/(m/s)  PxUpperLimitTransitionRegionWidth=1e-4  PxUpperLimitTransitionRegionWidthUnits=m  PxPositionTargetSpecify=off  PxPositionTargetPriority=High  PxPositionTargetValue=0  PxPositionTargetValueUnits=m  PxVelocityTargetSpecify=off  PxVelocityTargetPriority=High  PxVelocityTargetValue=0  PxVelocityTargetValueUnits=m/s  PyEquilibriumPosition=0  PyEquilibriumPositionUnits=m  PySpringStiffness=0  PySpringStiffnessUnits=N/m  PyDampingCoefficient=0  PyDampingCoefficientUnits=N/(m/s)  PyTorqueActuationMode=InputTorque  PyMotionActuationMode=ComputedMotion  PySensePosition=on  PySenseVelocity=on  PySenseAcceleration=off  PySenseTorqueForce=off  PySenseLowerLimitTorqueForce=off  PySenseUpperLimitTorqueForce=off  PyLowerLimitSpecify=off  PyLowerLimitBound=-1  PyLowerLimitBoundUnits=m  PyLowerLimitStiffness=1e6  PyLowerLimitStiffnessUnits=N/m  PyLowerLimitDamping=1e3  PyLowerLimitDampingUnits=N/(m/s)  PyLowerLimitTransitionRegionWidth=1e-4  PyLowerLimitTransitionRegionWidthUnits=m  PyUpperLimitSpecify=off  PyUpperLimitBound=1  PyUpperLimitBoundUnits=m  PyUpperLimitStiffness=1e6  PyUpperLimitStiffnessUnits=N/m  PyUpperLimitDamping=1e3  PyUpperLimitDampingUnits=N/(m/s)  PyUpperLimitTransitionRegionWidth=1e-4  PyUpperLimitTransitionRegionWidthUnits=m  PyPositionTargetSpecify=off  PyPositionTargetPriority=High  PyPositionTargetValue=0  PyPositionTargetValueUnits=m  PyVelocityTargetSpecify=off  PyVelocityTargetPriority=High  PyVelocityTargetValue=0  PyVelocityTargetValueUnits=m/s  PzEquilibriumPosition=0  PzEquilibriumPositionUnits=m  PzSpringStiffness=0  PzSpringStiffnessUnits=N/m  PzDampingCoefficient=0  PzDampingCoefficientUnits=N/(m/s)  PzTorqueActuationMode=InputTorque  PzMotionActuationMode=ComputedMotion  PzSensePosition=on  PzSenseVelocity=on  PzSenseAcceleration=off  PzSenseTorqueForce=off  PzSenseLowerLimitTorqueForce=off  PzSenseUpperLimitTorqueForce=off  PzLowerLimitSpecify=off  PzLowerLimitBound=-1  PzLowerLimitBoundUnits=m  PzLowerLimitStiffness=1e6  PzLowerLimitStiffnessUnits=N/m  PzLowerLimitDamping=1e3  PzLowerLimitDampingUnits=N/(m/s)  PzLowerLimitTransitionRegionWidth=1e-4  PzLowerLimitTransitionRegionWidthUnits=m  PzUpperLimitSpecify=off  PzUpperLimitBound=1  PzUpperLimitBoundUnits=m  PzUpperLimitStiffness=1e6  PzUpperLimitStiffnessUnits=N/m  PzUpperLimitDamping=1e3  PzUpperLimitDampingUnits=N/(m/s)  PzUpperLimitTransitionRegionWidth=1e-4  PzUpperLimitTransitionRegionWidthUnits=m  PzPositionTargetSpecify=off  PzPositionTargetPriority=High  PzPositionTargetValue=0  PzPositionTargetValueUnits=m  PzVelocityTargetSpecify=off  PzVelocityTargetPriority=High  PzVelocityTargetValue=0  PzVelocityTargetValueUnits=m/s
  Constant : Constant  Value=[q0_ang_deg]  VectorParams1D=off
  Display : Display
  MEAS_ANG : Subsystem
  MEAS_XYZ : Subsystem
  Mechanism Configuration : sm_lib/Utilities/Mechanism Configuration  UniformGravity=Constant  GravityVector=[0 0 -9.80665]  GravityUnits=m/s^2  LinearizationDelta=0.001  JointModeTransitionNonlinearIterations=2
  PEND : sm_lib/Body Elements/Brick Solid  GraphicAmbientColor=[0.15 0.15 0.15 1.0]  BasedOnType=Mass  BrickDimensions=[Lx, Ly, Lz]  BrickDimensionUnits=m  CenterOfMass=[0 0 0]  CenterOfMassUnits=m  GraphicDiffuseColor=[1.0 0.6 0.2]  Density=1000  DensityUnits=kg/(m^3)  DoExposeReferenceFrame=on  GraphicEmissiveColor=[0.0 0.0 0.0 1.0]  ExportEntireGeometry=off  SerializedFrames=<Frames/>  MarkerShape=Sphere  MarkerSize=10  GraphicType=FromGeometry  InertiaType=CalculateFromGeometry  Mass=m_pend  MassUnits=kg  MomentsOfInertia=[1 1 1]  MomentsOfInertiaUnits=kg*m^2  GraphicOpacity=1.0  ProductsOfInertia=[0 0 0]  ProductsOfInertiaUnits=kg*m^2  GraphicShininess=75  GraphicSpecularColor=[0.5 0.5 0.5 1.0]  GraphicVisPropType=SimpleVisualProperties
  PS-Simulink Converter : nesl_utility/PS-Simulink Converter  PhysicalDomain=network_engine_domain  SubClassName=ps_output  LeftPortType=input  RightPortType=output  PseudoPeriodic=off  Frequencies=[]  Unit=m  AffineConversion=off
      settings: SourceProductBaseCode=PW,SS
  PS-Simulink Converter1 : nesl_utility/PS-Simulink Converter  PhysicalDomain=network_engine_domain  SubClassName=ps_output  LeftPortType=input  RightPortType=output  PseudoPeriodic=off  Frequencies=[]  Unit=m  AffineConversion=off
      settings: SourceProductBaseCode=PW,SS
  PS-Simulink Converter2 : nesl_utility/PS-Simulink Converter  PhysicalDomain=network_engine_domain  SubClassName=ps_output  LeftPortType=input  RightPortType=output  PseudoPeriodic=off  Frequencies=[]  Unit=m  AffineConversion=off
      settings: SourceProductBaseCode=PW,SS
  PS-Simulink Converter3 : nesl_utility/PS-Simulink Converter  PhysicalDomain=network_engine_domain  SubClassName=ps_output  LeftPortType=input  RightPortType=output  PseudoPeriodic=off  Frequencies=[]  Unit=m/s  AffineConversion=off
      settings: SourceProductBaseCode=PW,SS
  PS-Simulink Converter4 : nesl_utility/PS-Simulink Converter  PhysicalDomain=network_engine_domain  SubClassName=ps_output  LeftPortType=input  RightPortType=output  PseudoPeriodic=off  Frequencies=[]  Unit=m/s  AffineConversion=off
      settings: SourceProductBaseCode=PW,SS
  PS-Simulink Converter5 : nesl_utility/PS-Simulink Converter  PhysicalDomain=network_engine_domain  SubClassName=ps_output  LeftPortType=input  RightPortType=output  PseudoPeriodic=off  Frequencies=[]  Unit=m/s  AffineConversion=off
      settings: SourceProductBaseCode=PW,SS
  RT_Set_SPH : sm_lib/Frames and Transforms/Rigid Transform  TranslationMethod=StandardAxis  TranslationStandardOffset=Tv_Z  TranslationLengthUnit=m  TranslationStandardAxis=+Z  TranslationCartesianOffset=[0 0 0]  TranslationROffset=0  TranslationROffsetUnits=m  TranslationZOffset=0  TranslationZOffsetUnits=m  TranslationThetaOffset=0  TranslationThetaOffsetUnits=deg  RotationMethod=None  RotationAngleUnits=deg  RotationStandardAxis=+Z  RotationAngle=0  RotationArbitraryAxis=[0 0 1]  FollAlignAxisA=+X  BaseAlignAxisA=+Y  FollAlignAxisB=+Y  BaseAlignAxisB=+Z  RotationSequenceAxes=FollowerAxes  RotationSequence=XYX  RotationSequenceAngles=[0 0 0]  RotationSequenceAnglesUnits=deg  RotationMatrix=[1 0 0; 0 1 0; 0 0 1]
  RT_topendCM : sm_lib/Frames and Transforms/Rigid Transform  TranslationMethod=StandardAxis  TranslationStandardOffset=Lz/2  TranslationLengthUnit=m  TranslationStandardAxis=+Z  TranslationCartesianOffset=[0 0 0]  TranslationROffset=0  TranslationROffsetUnits=m  TranslationZOffset=0  TranslationZOffsetUnits=m  TranslationThetaOffset=0  TranslationThetaOffsetUnits=deg  RotationMethod=None  RotationAngleUnits=deg  RotationStandardAxis=+Z  RotationAngle=0  RotationArbitraryAxis=[0 0 1]  FollAlignAxisA=+X  BaseAlignAxisA=+Y  FollAlignAxisB=+Y  BaseAlignAxisB=+Z  RotationSequenceAxes=FollowerAxes  RotationSequence=XYX  RotationSequenceAngles=[0 0 0]  RotationSequenceAnglesUnits=deg  RotationMatrix=[1 0 0; 0 1 0; 0 0 1]
  Simulink-PS Converter : nesl_utility/Simulink-PS Converter  PhysicalDomain=network_engine_domain  SubClassName=ps_input  LeftPortType=input  RightPortType=output  PseudoPeriodic=off  Frequencies=[]  NoiseDistribution=none  NoiseParameters=[]  Unit=N  AffineConversion=off  FilteringAndDerivatives=zero  SimscapeFilterOrder=1  InputFilterTimeConstant=0.001  UdotUserProvided=1
      settings: SourceProductBaseCode=PW,SS
  Simulink-PS Converter1 : nesl_utility/Simulink-PS Converter  PhysicalDomain=network_engine_domain  SubClassName=ps_input  LeftPortType=input  RightPortType=output  PseudoPeriodic=off  Frequencies=[]  NoiseDistribution=none  NoiseParameters=[]  Unit=N  AffineConversion=off  FilteringAndDerivatives=zero  SimscapeFilterOrder=1  InputFilterTimeConstant=0.001  UdotUserProvided=1
      settings: SourceProductBaseCode=PW,SS
  Simulink-PS Converter2 : nesl_utility/Simulink-PS Converter  PhysicalDomain=network_engine_domain  SubClassName=ps_input  LeftPortType=input  RightPortType=output  PseudoPeriodic=off  Frequencies=[]  NoiseDistribution=none  NoiseParameters=[]  Unit=N  AffineConversion=off  FilteringAndDerivatives=zero  SimscapeFilterOrder=1  InputFilterTimeConstant=0.001  UdotUserProvided=1
      settings: SourceProductBaseCode=PW,SS
  Solver Configuration : nesl_utility/Solver Configuration  PhysicalDomain=network_engine_domain  SubClassName=solver  LeftPortType=input  RightPortType=generic  Tones=[]  Harmonics=[]  SimulateNoise=off  Profile=off  UseLocalSampling=off  EnableSwitchedLinearOptims=on  FrequencyDomain=off  UseCCode=off  RelTol=0.001  AbsTol=1e-06  MinStep=1e-09  ToWorkspace=off  RevertToSquareIcSolve=off  NumHomotopyIterations=100  PhasorMode=off  PhasorModeNumHarmonics=1  DoDC=off  ResidualTolerance=1e-09  UseLocalSolver=off  LocalSolverChoice=NE_BACKWARD_EULER_ADVANCER  LocalSolverSampleTime=0.001  DoFixedCost=off  MaxNonlinIter=3  MaxModeIter=2  ComputeImpulses=off  ImpulseIterations=2  LinearAlgebra=Sparse  EquationFormulation=NE_TIME_EF  DelaysMemoryBudget=1024  AutomaticFiltering=on  FilteringTimeConstant=0.001  PartitionStorageMethod=AS_NEEDED  PartitionMemoryBudget=1024  PartitionMethod=FAST
      settings: SourceProductBaseCode=PW,SS
  Spherical Joint : sm_lib/Joints/Spherical Joint  JointMode=Normal  SenseConstraintForce=off  SenseConstraintForceX=off  SenseConstraintForceY=off  SenseConstraintForceZ=off  SenseConstraintTorque=off  SenseConstraintTorqueX=off  SenseConstraintTorqueY=off  SenseConstraintTorqueZ=off  SenseTotalForce=off  SenseTotalForceX=off  SenseTotalForceY=off  SenseTotalForceZ=off  SenseTotalTorque=off  SenseTotalTorqueX=off  SenseTotalTorqueY=off  SenseTotalTorqueZ=off  CompositeWrenchDir=FollowerOnBase  CompositeWrenchFrame=BaseFrame  DefPosRotationMethod=None  DefPosRotationAngleUnits=deg  DefPosRotationStandardAxis=+Z  DefPosRotationAngle=0.0  DefPosRotationArbitraryAxis=[0 0 1]  DefPosFollAlignAxisA=+X  DefPosBaseAlignAxisA=+Y  DefPosFollAlignAxisB=+Y  DefPosBaseAlignAxisB=+Z  DefPosRotationSequenceAxes=FollowerAxes  DefPosRotationSequence=XYX  DefPosRotationSequenceAngles=[0 0 0]  DefPosRotationSequenceAnglesUnits=deg  DefPosRotationMatrix=[1 0 0; 0 1 0; 0 0 1]  EqPosRotationMethod=None  EqPosRotationAngleUnits=deg  EqPosRotationStandardAxis=+Z  EqPosRotationAngle=0.0  EqPosRotationArbitraryAxis=[0 0 1]  EqPosFollAlignAxisA=+X  EqPosBaseAlignAxisA=+Y  EqPosFollAlignAxisB=+Y  EqPosBaseAlignAxisB=+Z  EqPosRotationSequenceAxes=FollowerAxes  EqPosRotationSequence=XYX  EqPosRotationSequenceAngles=[0 0 0]  EqPosRotationSequenceAnglesUnits=deg  EqPosRotationMatrix=[1 0 0; 0 1 0; 0 0 1]  SpringStiffness=0  SpringStiffnessUnits=N*m/deg  DampingCoefficient=0  DampingCoefficientUnits=N*m/(deg/s)  ActuateTorqueX=off  ActuateTorqueY=off  ActuateTorqueZ=off  ActuateTorque=off  TorqueActuationMode=NoTorque  MotionActuationMode=ComputedMotion  ActuationFrame=BaseFrame  SensePosition=off  SenseVelocityX=off  SenseVelocityY=off  SenseVelocityZ=off  SenseVelocity=off  SenseAccelerationX=off  SenseAccelerationY=off  SenseAccelerationZ=off  SenseAcceleration=off  SenseTorqueX=off  SenseTorqueY=off  SenseTorqueZ=off  SenseTorqueForce=off  SenseLowerLimitTorqueMag=off  SenseUpperLimitTorqueMag=off  SensingFrame=BaseFrame  LowerLimitSpecify=off  LowerLimitBound=15  LowerLimitBoundUnits=deg  LowerLimitStiffness=1e4  LowerLimitStiffnessUnits=N*m/deg  LowerLimitDamping=10  LowerLimitDampingUnits=N*m/(deg/s)  LowerLimitTransitionRegionWidth=0.1  LowerLimitTransitionRegionWidthUnits=deg  UpperLimitSpecify=off  UpperLimitBound=45  UpperLimitBoundUnits=deg  UpperLimitStiffness=1e4  UpperLimitStiffnessUnits=N*m/deg  UpperLimitDamping=10  UpperLimitDampingUnits=N*m/(deg/s)  UpperLimitTransitionRegionWidth=0.1  UpperLimitTransitionRegionWidthUnits=deg  PositionTargetRotationMethod=RotationSequence  PositionTargetRotationAngleUnits=deg  PositionTargetRotationStandardAxis=+Z  PositionTargetRotationAngle=0.0  PositionTargetRotationArbitraryAxis=[0 0 1]  PositionTargetFollAlignAxisA=+X  PositionTargetBaseAlignAxisA=+Y  PositionTargetFollAlignAxisB=+Y  PositionTargetBaseAlignAxisB=+Z  PositionTargetRotationSequenceAxes=FollowerAxes  PositionTargetRotationSequence=ZYX  PositionTargetRotationSequenceAngles=[q0_ang_deg]  PositionTargetRotationSequenceAnglesUnits=deg  PositionTargetRotationMatrix=[1 0 0; 0 1 0; 0 0 1]  PositionTargetSpecify=on  PositionTargetPriority=High  VelocityTargetValue=[q0_dot_and_deg]  VelocityTargetValueUnits=deg/s  VelocityTargetSpecify=on  VelocityTargetPriority=High  VelocityTargetInFollowerFrame=on
      settings: AttributesFormatString=|
      | %<PositionTargetRotationSequenceAnglesUnits>
      | %<PositionTargetRotationSequenceAngles>
      | %<PositionTargetRotationSequence>
  World Frame : sm_lib/Frames and Transforms/World Frame
  crwate_MeBUS : Subsystem
  MeBus : Outport  VectorParamsAs1DForOutWhenUnconnected=off
  wires:
  Fg_z/1 -> Simulink-PS Converter/1
  Fg_y/1 -> Simulink-PS Converter2/1
  Fg_x/1 -> Simulink-PS Converter1/1
  crwate_MeBUS/1(MEAS_BUS) -> [MeBus]
  MEAS_XYZ/1(MeBus) -> MEAS_ANG/1(IN_MeBus)
  PS-Simulink Converter2/1 -> MEAS_XYZ/5(pz)
  PS-Simulink Converter1/1 -> MEAS_XYZ/3(py)
  PS-Simulink Converter3/1 -> MEAS_XYZ/2(vx)
  PS-Simulink Converter/1 -> MEAS_XYZ/1(px)
  PS-Simulink Converter4/1 -> MEAS_XYZ/4(vy)
  PS-Simulink Converter5/1 -> MEAS_XYZ/6(vz)
  [MeBus] -> MEAS_XYZ/7(IN_MeBus)
  MEAS_ANG/1(MeBus) -> MeBus/1
  Constant/1 -> Display/1
  connections:
  Spherical Joint/LConn1 -- MEAS_ANG/LConn1 -- RT_Set_SPH/RConn1
  Mechanism Configuration/RConn1 -- Solver Configuration/RConn1 -- World Frame/RConn1 -- Cartesian Joint/LConn1
  RT_topendCM/LConn1 -- MEAS_ANG/RConn1 -- Spherical Joint/RConn1
  CART/RConn1 -- RT_Set_SPH/LConn1 -- Cartesian Joint/RConn1
  RT_topendCM/RConn1 -- PEND/RConn1
  Simulink-PS Converter/RConn1 -- Cartesian Joint/LConn4
  Simulink-PS Converter2/RConn1 -- Cartesian Joint/LConn3
  Simulink-PS Converter1/RConn1 -- Cartesian Joint/LConn2
  PS-Simulink Converter2/LConn1 -- Cartesian Joint/RConn6
  Cartesian Joint/RConn4 -- PS-Simulink Converter1/LConn1
  Cartesian Joint/RConn2 -- PS-Simulink Converter/LConn1
  Cartesian Joint/RConn7 -- PS-Simulink Converter5/LConn1
  Cartesian Joint/RConn5 -- PS-Simulink Converter4/LConn1
  Cartesian Joint/RConn3 -- PS-Simulink Converter3/LConn1

== system bh_3d_pend_sim_CONTROLLED/a_circle/Signal Builder ==
  Demux : Demux  Tag=STV Demux  Outputs=2
      settings: DisplayOption=none
  FromWs : FromWorkspace  Tag=STV FromWs  VariableName=tuvar
      SigBuilderData=|
      | common.afterFinalStr = 'Extrapolate'
      | common.sampleTime = 0
      | dataSet.timeRange = [0 22]
      | dataSet.name = 'Group 1'
      | sbobj.Groups.Name = 'Group 1'
      | sbobj.Groups.Signals(1).Name = 'Signal 1'
      | sbobj.Groups.Signals(1).XData = [0 7.95 7.95 22]
      | sbobj.Groups.Signals(1).YData = [0 0 1.99 1.98]
      | sbobj.Groups.Signals(2).Name = 'Signal 2'
      | sbobj.Groups.Signals(2).XData = [0 12 16 22]
      | sbobj.Groups.Signals(2).YData = [0 0 1 1]
      | sbobj.Groups.TimeRange = [0 22]
  Signal 1 : Outport  Tag=STV Outport  VectorParamsAs1DForOutWhenUnconnected=off
  Signal 2 : Outport  Tag=STV Outport  Port=2  VectorParamsAs1DForOutWhenUnconnected=off
  wires:
  Demux/1 -> Signal 1/1
  FromWs/1 -> Demux/1
  Demux/2 -> Signal 2/1

== system bh_3d_pend_sim_CONTROLLED/a_circle/Subsystem ==
  RPS : Inport
  Constant : Constant  Value=2*pi
  Product : Product  Inputs=**
  w_rad_psec : Outport  VectorParamsAs1DForOutWhenUnconnected=off
  wires:
  Constant/1 -> Product/2
  RPS/1 -> Product/1
  Product/1 -> w_rad_psec/1

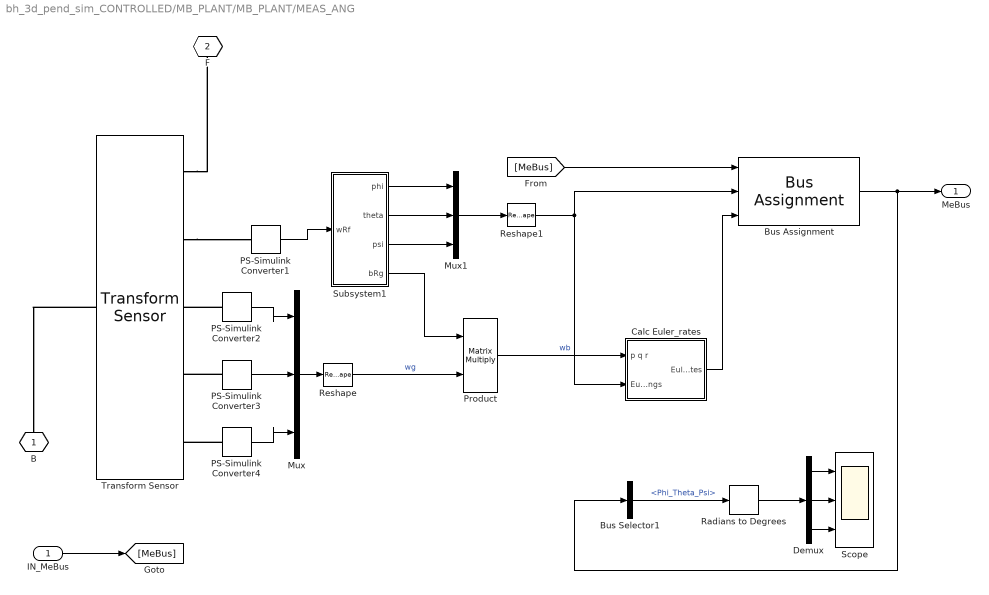
== system bh_3d_pend_sim_CONTROLLED/MB_PLANT/MB_PLANT/MEAS_ANG ==
  IN_MeBus : Inport
  Bus Assignment : BusAssignment  AssignedSignals=Phi_Theta_Psi,DOT_Phi_Theta_Psi
  Bus Selector1 : BusSelector  OutputSignals=Phi_Theta_Psi
  Calc Euler_rates : Subsystem
  Demux : Demux  Outputs=3
  Mux : Mux  Inputs=3
  Mux1 : Mux  Inputs=3
  PS-Simulink Converter1 : nesl_utility/PS-Simulink Converter  PhysicalDomain=network_engine_domain  SubClassName=ps_output  LeftPortType=input  RightPortType=output  PseudoPeriodic=off  Frequencies=[]  Unit=1  AffineConversion=off
      settings: SourceProductBaseCode=PW,SS
  PS-Simulink Converter2 : nesl_utility/PS-Simulink Converter  PhysicalDomain=network_engine_domain  SubClassName=ps_output  LeftPortType=input  RightPortType=output  PseudoPeriodic=off  Frequencies=[]  Unit=rad/s  AffineConversion=off
      settings: SourceProductBaseCode=PW,SS
  PS-Simulink Converter3 : nesl_utility/PS-Simulink Converter  PhysicalDomain=network_engine_domain  SubClassName=ps_output  LeftPortType=input  RightPortType=output  PseudoPeriodic=off  Frequencies=[]  Unit=rad/s  AffineConversion=off
      settings: SourceProductBaseCode=PW,SS
  PS-Simulink Converter4 : nesl_utility/PS-Simulink Converter  PhysicalDomain=network_engine_domain  SubClassName=ps_output  LeftPortType=input  RightPortType=output  PseudoPeriodic=off  Frequencies=[]  Unit=rad/s  AffineConversion=off
      settings: SourceProductBaseCode=PW,SS
  Product : Product  Multiplication=Matrix(*)
  Radians to Degrees : simulink_extras/Transformations/Radians to Degrees
  Reshape : Reshape  OutputDimensionality=Column vector (2-D)
  Reshape1 : Reshape  OutputDimensionality=Column vector (2-D)
  Scope : Scope  NumInputPorts=3
  Subsystem1 : Subsystem
  Transform Sensor : sm_lib/Frames and Transforms/Transform Sensor  MeasurementFrame=World  SenseAngle=off  SenseAxis=off  SenseAngle1=off  SenseAngle2=off  SenseAngle3=off  SenseQ=off  SenseR=on  SenseOmegaX=on  SenseOmegaY=on  SenseOmegaZ=on  SenseOmega1=off  SenseOmega2=off  SenseOmega3=off  SenseQDot=off  SenseRDot=off  SenseAlphaX=off  SenseAlphaY=off  SenseAlphaZ=off  SenseAlpha1=off  SenseAlpha2=off  SenseAlpha3=off  SenseQDDot=off  SenseRDDot=off  SenseX=off  SenseY=off  SenseZ=off  SenseRad=off  SenseAzim=off  SenseDist=off  SenseInc=off  SenseXDot=off  SenseYDot=off  SenseZDot=off  SenseRadDot=off  SenseAzimDot=off  SenseDistDot=off  SenseIncDot=off  SenseXDDot=off  SenseYDDot=off  SenseZDDot=off  SenseRadDDot=off  SenseAzimDDot=off  SenseDistDDot=off  SenseIncDDot=off
      settings: AttributesFormatString=MeasComponentFrame = %<MeasurementFrame>
  B : PMIOPort  Side=Left
  F : PMIOPort  Port=2  Side=Right
  MeBus : Outport  VectorParamsAs1DForOutWhenUnconnected=off
  wires:
  PS-Simulink Converter1/1 -> Subsystem1/1(wRf)
  Subsystem1/1(phi) -> Mux1/1
  Subsystem1/3(psi) -> Mux1/3
  PS-Simulink Converter2/1 -> Mux/1
  PS-Simulink Converter3/1 -> Mux/2
  PS-Simulink Converter4/1 -> Mux/3
  Mux/1 -> Reshape/1
  Subsystem1/4(bRg) -> Product/1
  Reshape/1 -> Product/2  "wg"
  Product/1 -> Calc Euler_rates/1("p q r ")  "wb"
  Subsystem1/2(theta) -> Mux1/2
  IN_MeBus/1 -> [MeBus]
  Mux1/1 -> Reshape1/1
  [MeBus] -> Bus Assignment/1
  Reshape1/1 -> Bus Assignment/2, Calc Euler_rates/2(Euler_angs)
  Calc Euler_rates/1(Euler_rates) -> Bus Assignment/3
  Bus Assignment/1 -> Bus Selector1/1, MeBus/1
  Bus Selector1/1 -> Radians to Degrees/1  "<Phi_Theta_Psi>"
  Demux/1 -> Scope/1
  Demux/2 -> Scope/2
  Demux/3 -> Scope/3
  Radians to Degrees/1 -> Demux/1
  connections:
  PS-Simulink Converter2/LConn1 -- Transform Sensor/RConn3
  PS-Simulink Converter4/LConn1 -- Transform Sensor/RConn5
  PS-Simulink Converter3/LConn1 -- Transform Sensor/RConn4
  Transform Sensor/LConn1 -- B/RConn1
  Transform Sensor/RConn1 -- F/RConn1
  Transform Sensor/RConn2 -- PS-Simulink Converter1/LConn1

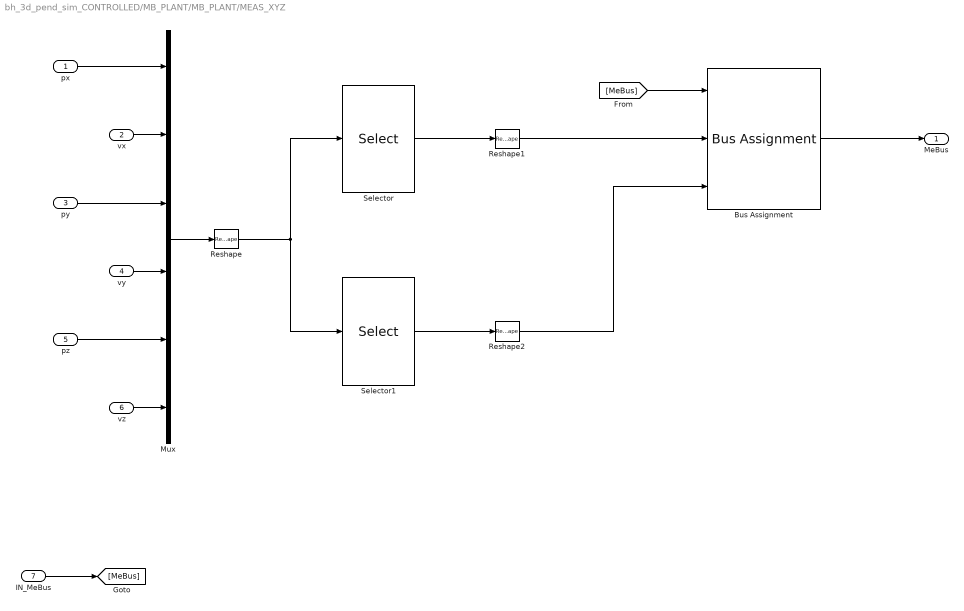
== system bh_3d_pend_sim_CONTROLLED/MB_PLANT/MB_PLANT/MEAS_XYZ ==
  px : Inport
  vx : Inport  Port=2
  py : Inport  Port=3
  vy : Inport  Port=4
  pz : Inport  Port=5
  vz : Inport  Port=6
  IN_MeBus : Inport  Port=7
  Bus Assignment : BusAssignment  AssignedSignals=XYZ,DOT_XYZ
  Mux : Mux  Inputs=6
  Reshape : Reshape  OutputDimensionality=Column vector (2-D)
  Reshape1 : Reshape  OutputDimensionality=Column vector (2-D)
  Reshape2 : Reshape  OutputDimensionality=Column vector (2-D)
  Selector : Selector  InputPortWidth=6  IndexOptions=Index vector (dialog)  Indices=[1 3 5]  OutputSizes=1
  Selector1 : Selector  InputPortWidth=6  IndexOptions=Index vector (dialog)  Indices=[2 4 6]  OutputSizes=1
  MeBus : Outport  VectorParamsAs1DForOutWhenUnconnected=off
  wires:
  vz/1 -> Mux/6
  pz/1 -> Mux/5
  vy/1 -> Mux/4
  py/1 -> Mux/3
  vx/1 -> Mux/2
  px/1 -> Mux/1
  Mux/1 -> Reshape/1
  Reshape/1 -> Selector1/1, Selector/1
  Selector/1 -> Reshape1/1
  Selector1/1 -> Reshape2/1
  IN_MeBus/1 -> [MeBus]
  [MeBus] -> Bus Assignment/1
  Bus Assignment/1 -> MeBus/1
  Reshape1/1 -> Bus Assignment/2
  Reshape2/1 -> Bus Assignment/3

== system bh_3d_pend_sim_CONTROLLED/MB_PLANT/MB_PLANT/crwate_MeBUS ==
  Bus Creator : BusCreator  Inputs=4
  Constant{1..4} (4 alike) : Constant  Value=[0,0,0]
  Reshape{,1..3} (4 alike) : Reshape  OutputDimensionality=Column vector (2-D)
  MEAS_BUS : Outport  VectorParamsAs1DForOutWhenUnconnected=off
  wires:
  Reshape/1 -> Bus Creator/1  "Phi_Theta_Psi"
  Reshape1/1 -> Bus Creator/2  "DOT_Phi_Theta_Psi"
  Reshape2/1 -> Bus Creator/3  "XYZ"
  Reshape3/1 -> Bus Creator/4  "DOT_XYZ"
  Constant1/1 -> Reshape/1
  Constant2/1 -> Reshape1/1
  Constant3/1 -> Reshape2/1
  Constant4/1 -> Reshape3/1
  Bus Creator/1 -> MEAS_BUS/1

== system bh_3d_pend_sim_CONTROLLED/MB_PLANT/MB_PLANT/MEAS_ANG/Calc Euler_rates ==
  "p q r " : Inport
  Euler_angs : Inport  Port=2
  Demux1 : Demux  Outputs=3
  Demux2 : Demux  Outputs=3
  Demux3 : Demux  Outputs=3
  Mux1 : Mux  Inputs=3
  Reshape1 : Reshape  OutputDimensionality=Column vector (2-D)
  Reshape2 : Reshape  OutputDimensionality=Column vector (2-D)
  Terminator : Terminator
  my_euler_rates : MATLAB Function  TreatAsAtomicUnit=on
  Euler_rates : Outport  VectorParamsAs1DForOutWhenUnconnected=off
  wires:
  Reshape1/1 -> Demux3/1  "wb"
  my_euler_rates/1(euler_rates) -> Demux2/1  "euler_rates"
  Demux2/3 -> Mux1/3  "psidot_X3_roll"
  Demux2/2 -> Mux1/2  "thetadot_Y2_pitch"
  Demux2/1 -> Mux1/1  "phidot_Z1_yaw"
  Reshape2/1 -> Euler_rates/1
  Mux1/1 -> Reshape2/1
  Demux3/3 -> my_euler_rates/5(r)
  Demux3/2 -> my_euler_rates/4(q)
  Demux3/1 -> my_euler_rates/3(p)
  Euler_angs/1 -> Demux1/1
  "p q r "/1 -> Reshape1/1
  Demux1/2 -> my_euler_rates/1(theta)  "theta"
  Demux1/1 -> Terminator/1  "phi"
  Demux1/3 -> my_euler_rates/2(psi)  "psi"

== system bh_3d_pend_sim_CONTROLLED/MB_PLANT/MB_PLANT/MEAS_ANG/Subsystem1 ==
  wRf : Inport
  Gain : Gain
  MATLAB Function : MATLAB Function  TreatAsAtomicUnit=on
  Math Function : Math  Operator=transpose  SignedPower=on  SaturateOnIntegerOverflow=on
  phi : Outport  VectorParamsAs1DForOutWhenUnconnected=off
  theta : Outport  Port=2  VectorParamsAs1DForOutWhenUnconnected=off
  psi : Outport  Port=3  VectorParamsAs1DForOutWhenUnconnected=off
  bRg : Outport  Port=4  VectorParamsAs1DForOutWhenUnconnected=off
  wires:
  wRf/1 -> Gain/1
  Gain/1 -> Math Function/1  "gRb"
  Math Function/1 -> bRg/1, MATLAB Function/1(bRg)  "bRg"
  MATLAB Function/1(phi) -> phi/1
  MATLAB Function/2(theta) -> theta/1
  MATLAB Function/3(psi) -> psi/1
